simulink model "trajectory_p"  (R2018b)
settings: Solver=VariableStepAuto  StartTime=0.0  StopTime=60  RelTol=1e-3
values from neighbouring files (symbols this model uses):
  bike =     [bike.mat]    (also in modelconfig.mat)
  controller =     [modelconfig.mat]
  model_settings =     [modelconfig.mat]
  parameters =     [modelconfig.mat]
  state_space =     [modelconfig.mat]
undefined symbols (not defined in the file or in its folder): Continuous, Noise, observer, Time
libraries: simulink x4, dspindex x3, ctrlSharedLib x1
(part 2 of 2)

== matlab function trajectory_p/Trajectory/MATLAB Function ==
  data: t input; v output; t_case input; v0 input
function v = fcn(t,t_case, v0)


switch t_case
    case 1
        v = v0;
    case 2
        if t < 15
            v = v0;
        elseif t < 35
            v = v0 - v0/20*(t-15);
        else
            v = 0;
        end
    case 3
        if t < 5
            v = v0;
        elseif t < 15
            v = v0 + v0/20*(t-5);
        elseif t < 20
            v = v0 + v0/2;
        elseif t < 30
            v = 1.5*v0 - v0/20*(t-20);
        else
            v = v0;
        end
    case 4
        if t < 5
            v = v0;
        elseif t < 15
            v = v0 + v0/20*(t-5);
        elseif t < 20
            v = v0 + v0/2;
        elseif t < 40
            v = 1.5*v0 - v0/20*(t-20);
        elseif t < 45
            v = 0.5*v0;
        elseif t < 55
            v = 0.5*v0 - v0/20*(t-45);
        else
            v = 0;
        end
    case 5
        if t < 5
            v = v0;
        elseif t < 9
            v = v0 - v0/40*(t-5);
        else
            v = v0 - v0/40*(4);
        end
    case 6
        if t < 10
            v = v0 + v0/5*t;
        else
            v = 3*v0;
        end
    case 7
        if t < 5
            v = v0;
        elseif t < 10
            v = v0 + v0/5*(t-5);
        else
            v = 2*v0;
        end
    case 8
        v = 2; 
    otherwise
        v = v0;
end

== matlab function trajectory_p/Trajectory/Convert statespace to worldframe/Convert Statespace to World frame ==
  data: orientation_n input; delta input; Vel_BW output; velocity input
function Vel_BW   = fcn(orientation_n,delta,velocity)
% This converts the two variables delta and v from the statespace 
% [delta,ddelta,theta,dtheta,v] into global position coordinates.


% Shorten the inputnames
psi = orientation_n;
v = velocity;

L = 1.1; % L = bike.wheelbase;

% Forward kinematics from backwheel to frontwheel
H_BF = [1, 0, L;... % Might not be necessary
        0, 1, 0;...
        0, 0, 1];
% Forward kinematics from World frame to inner frame 
H_IG = [cos(psi),   sin(psi),   0;...
        -sin(psi),  cos(psi),   0;...
        0,          0,          1];    
    
Vel_FI = [   v;                  ...
            v*tan(-delta);       ...% The minus sign is just so that if the 
            1               ];      % angle is negative it should turn left 
                                    % Its estetics         
                               
VelBW = H_IG*Vel_FI;                % According to my math it should be
Vel_BW = VelBW(1:2);                % VelBW = H_IG/H_BF\Vel_FI, but results 
                                    % are odd

end

== matlab function trajectory_p/Monitor/Convert statespace to worldframe1/Convert Statespace to World frame ==
  data: orientation_n input; delta input; Vel_BW output; velocity input; Vel_FW output
function [Vel_BW,Vel_FW]  = fcn(orientation_n,delta,velocity)
% This converts the two variables delta and v from the statespace 
% [delta,ddelta,theta,dtheta,v] into global position coordinates.


% Shorten the inputnames
psi = orientation_n;
v = velocity;

L = 1.1; % L = bike.wheelbase;

% Forward kinematics from backwheel to frontwheel
H_BF = [1, 0, L;... % Might not be necessary
        0, 1, 0;...
        0, 0, 1];
% Forward kinematics from World frame to inner frame 
H_IG = [cos(psi),   sin(psi),   0;...
        -sin(psi),  cos(psi),   0;...
        0,          0,          1];    
    
Vel_FI = [   v;                  ...
            v*tan(-delta);       ...% The minus sign is just so that if the 
            1               ];      % angle is negative it should turn left 
                                    % Its estetics         
                               
VelBW = H_IG*H_BF\Vel_FI;                % According to my math it should be
Vel_BW = VelBW(1:2);                % VelBW = H_IG/H_BF\Vel_FI, but results 
VelFW = H_IG*Vel_FI;                                   % are odd
Vel_FW = VelFW(1:2);

end
